simulink model "fluidDynamicSurface_th"  (R2018b)
settings: Solver=VariableStepAuto  StartTime=0.0  StopTime=0  RelTol=1e-3
libraries: fluidDynamicSurface_cl x1
settings Model: Creator=mcobb  LastModifiedBy=mcobb

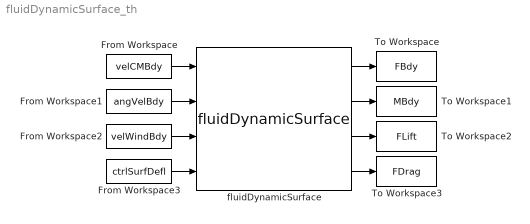
== system fluidDynamicSurface_th ==
  From Workspace : FromWorkspace  VariableName=velCMBdy  SampleTime=0
  From Workspace1 : FromWorkspace  VariableName=angVelBdy  SampleTime=0
  From Workspace2 : FromWorkspace  VariableName=velWindBdy  SampleTime=0
  From Workspace3 : FromWorkspace  VariableName=ctrlSurfDefl  SampleTime=0
  To Workspace : ToWorkspace  VariableName=FBdy  SaveFormat=Timeseries  SampleTime=-1
  To Workspace1 : ToWorkspace  VariableName=MBdy  SaveFormat=Timeseries  SampleTime=-1
  To Workspace2 : ToWorkspace  VariableName=FLift  SaveFormat=Timeseries  SampleTime=-1
  To Workspace3 : ToWorkspace  VariableName=FDrag  SaveFormat=Timeseries  SampleTime=-1
  fluidDynamicSurface : fluidDynamicSurface_cl/fluidDynamicSurface  refArea=refArea  aeroCentPosVecBdy=aeroCentPosVec  spanVec=spanUnitVec  chordVec=chordUnitVec
  wires:
  fluidDynamicSurface/2 -> To Workspace1/1
  fluidDynamicSurface/1 -> To Workspace/1
  From Workspace/1 -> fluidDynamicSurface/1
  From Workspace1/1 -> fluidDynamicSurface/2
  From Workspace2/1 -> fluidDynamicSurface/3
  From Workspace3/1 -> fluidDynamicSurface/4
  fluidDynamicSurface/3 -> To Workspace2/1
  fluidDynamicSurface/4 -> To Workspace3/1
